simulink model "Sodel_my_6dof_euler"  (R2017b)
settings: Solver=VariableStepAuto  StartTime=0.0  StopTime=Tsim  RelTol=0.01
values from neighbouring files (symbols this model uses):
  u1max = 25*pi/180    (= 0.436332312999)    [init.m]
  u1min = -25*pi/180    (= -0.436332312999)    [init.m]
  u2max = 10*pi/180    (= 0.174532925199)    [init.m]
  u2min = -25*pi/180    (= -0.436332312999)    [init.m]
  u3max = 30*pi/180    (= 0.523598775598)    [init.m]
  u3min = -30*pi/180    (= -0.523598775598)    [init.m]
  u4max = 10*pi/180    (= 0.174532925199)    [init.m]
  u4min = -0.5*pi/180    (= -0.00872664625997)    [init.m]
  u5max = 10*pi/180    (= 0.174532925199)    [init.m]
  u5min = -0.5*pi/180    (= -0.00872664625997)    [init.m]
  uu = [0; -0.1; 0; 0.0821; 0.0821]    [init.m]
  x0 = [100;0;0;0;0;0;0;0.1;0]    [init.m]
undefined symbols (not defined in the file or in its folder): Earth, sodel_6dof, WGS84
libraries: aerolibtransform2 x1, aerolibfltsims x1, shared6dof x1, dspnetwork x1
settings Model: Creator=Admin  LastModifiedBy=Admin
settings ConfigComp: CovHTMLOptions=-sRT=1 -sVT=0 -aTS=1 -bRG=1 -bTC=1 -hTR=1 -nFC=0 -nFD=1 -scm=1 -bcm=1 -xEv=0 -xEM=0

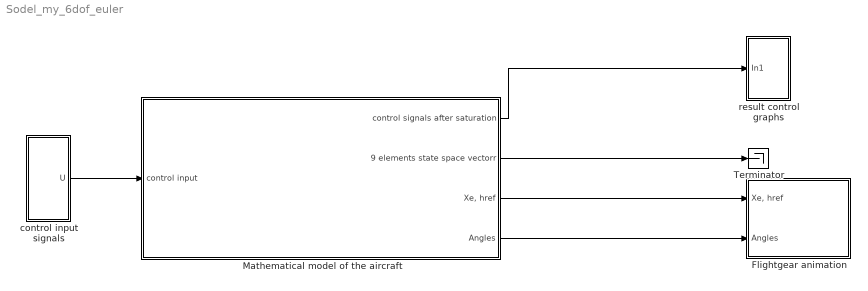
== system Sodel_my_6dof_euler ==
  Flightgear animation : Subsystem
  Mathematical model of the aircraft : Subsystem
  Terminator : Terminator
  control input signals : Subsystem
  result control graphs : Subsystem
  wires:
  control input signals/1(U) -> Mathematical model of the aircraft/1(control input)
  Mathematical model of the aircraft/1(control signals after saturation) -> result control graphs/1(In1)
  Mathematical model of the aircraft/2(9 elements state space vectorr) -> Terminator/1
  Mathematical model of the aircraft/3("Xe, href") -> Flightgear animation/1("Xe, href")
  Mathematical model of the aircraft/4(Angles) -> Flightgear animation/2(Angles)

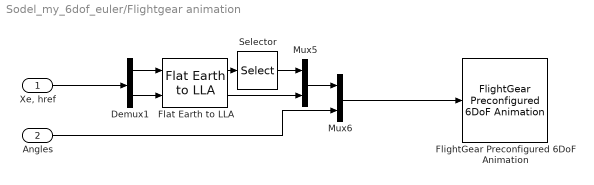
== system Sodel_my_6dof_euler/Flightgear animation ==
  "Xe, href" : Inport
  Angles : Inport  Port=2
  Demux1 : Demux  Outputs=2
  Flat Earth to LLA : aerolibtransform2/Flat Earth to LLA  units=Metric (MKS)  ptype=Earth (WGS84)  F=1/298.257223563  R=6378137  LL0=[37.6272 -122.3896]  psi=0
  FlightGear Preconfigured 6DoF Animation : aerolibfltsims/FlightGear Preconfigured 6DoF Animation  xFlightGearVersion=v2017.1  DestinationIpAddress=127.0.0.1  DestinationPort=5502  SampleTime=1/60
      settings: SourceProductName=Aerospace Blockset
  Mux5 : Mux  Inputs=2
  Mux6 : Mux  Inputs=2
  Selector : Selector  IndexMode=Zero-based  InputPortWidth=2  IndexOptions=Index vector (dialog)  Indices=[1 0]  OutputSizes=1
  wires:
  Mux6/1 -> FlightGear Preconfigured 6DoF Animation/1
  Angles/1 -> Mux6/2
  Demux1/2 -> Flat Earth to LLA/2
  "Xe, href"/1 -> Demux1/1
  Demux1/1 -> Flat Earth to LLA/1
  Flat Earth to LLA/1 -> Selector/1
  Flat Earth to LLA/2 -> Mux5/2
  Selector/1 -> Mux5/1
  Mux5/1 -> Mux6/1

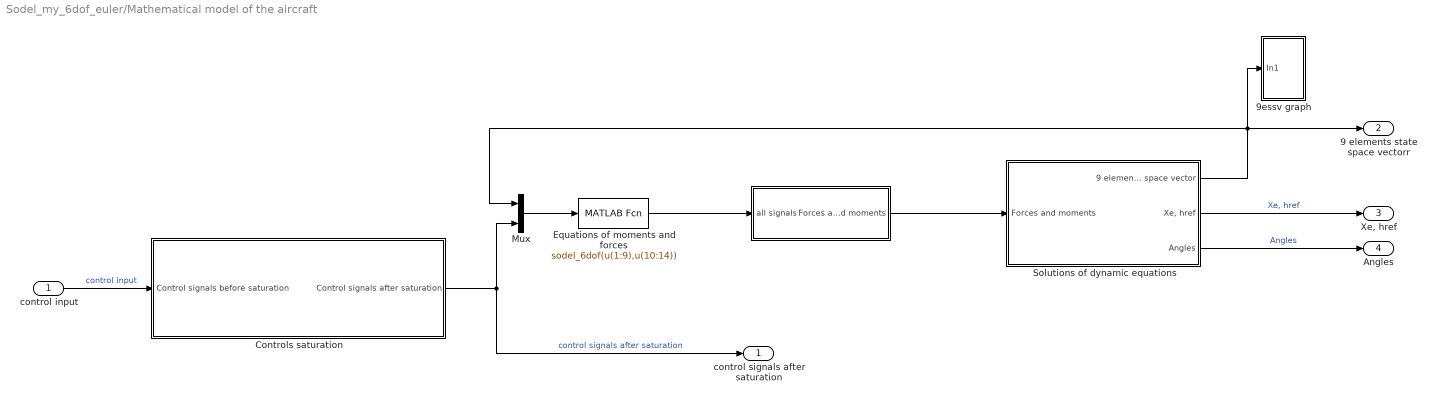
== system Sodel_my_6dof_euler/Mathematical model of the aircraft ==
  control input : Inport
  " " : Subsystem
  9essv graph : Subsystem
  Controls saturation : Subsystem
  Equations of moments and forces : MATLABFcn  MATLABFcn=sodel_6dof(u(1:9),u(10:14))
  Mux : Mux  Inputs=2
  Solutions of dynamic equations : Subsystem
  control signals after saturation : Outport
  9 elements state space vectorr : Outport  Port=2
  "Xe, href" : Outport  Port=3
  Angles : Outport  Port=4
  wires:
  Mux/1 -> Equations of moments and forces/1
  Solutions of dynamic equations/1(9 elements state space vector) -> 9essv graph/1(In1), Mux/1, 9 elements state space vectorr/1
  Solutions of dynamic equations/2("Xe, href") -> "Xe, href"/1  "Xe, href"
  Solutions of dynamic equations/3("Angles ") -> Angles/1  "Angles"
  Controls saturation/1(Control signals after saturation) -> control signals after saturation/1, Mux/2  "control signals after saturation"
  control input/1 -> Controls saturation/1(Control signals before saturation)  "control input"
  Equations of moments and forces/1 -> " "/1("all signals ")
  " "/1(Forces and moments) -> Solutions of dynamic equations/1(Forces and moments)

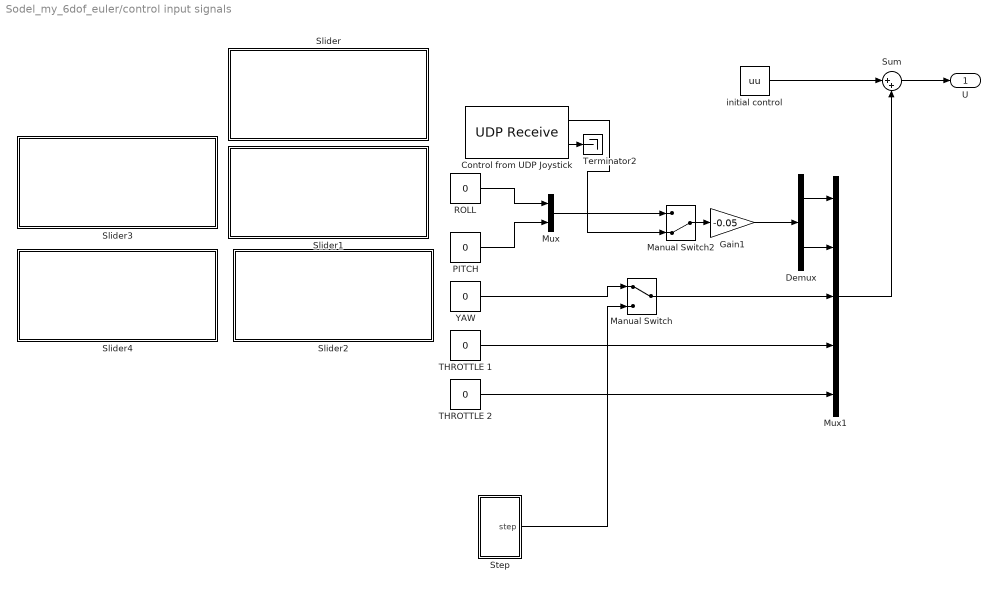
== system Sodel_my_6dof_euler/control input signals ==
  Control from UDP Joystick : dspnetwork/UDP Receive  localURL='0.0.0.0'  localPort=5005  remoteURL='0.0.0.0'  remotePort=-1  recvBufferSize=16  dims=2  signalDatatype=double  isVarSize=off  showBlockingTime=off  blockingTime=0  sampletime=1  blockPlatform=[]
      settings: SourceProductName=DSP System Toolbox  SourceProductBaseCode=DS
  Demux : Demux  Outputs=2
  Gain1 : Gain  Gain=-0.05
  Manual Switch : ManualSwitch
  Manual Switch2 : ManualSwitch  CurrentSetting=0
  Mux : Mux  Inputs=2
  Mux1 : Mux  Inputs=5
  PITCH : Constant  Value=0
  "ROLL " : Constant  Value=0
  Slider : Subsystem  DialogController=hmiCreateDDGDialog  IsWebBlock=on  mask(MWDashboardBlock){webBlockId=4142df3a-b1e0-45a1-953a-8fd48c9debc0, webBlockType=slider, ShowInLibBrowser=on, ShowInitialText=on, HMISrcModelName=Sodel_my_6dof_euler}
      mask prompts: webBlockId "WebBlock Id"; webBlockType "WebBlock Type"; HMISrcModelName "Source Model"
      mask help: SimulinkHMI:dialogs:SliderDialogDesc
      mask Help: helpview([docroot '/mapfiles/simulink.map'], 'hmi_slider')
      mask Display:
      | if strcmp(get_param(bdroot(gcb),'BlockDiagramType'), 'library')
      |     image([(matlabroot) '/toolbox/simulink/hmi/icons/Slider.png']);
      | end
  Slider1 : Subsystem  DialogController=hmiCreateDDGDialog  IsWebBlock=on  mask(MWDashboardBlock){webBlockId=67583dfa-0060-4976-b5ff-87e221de8104, webBlockType=slider, ShowInLibBrowser=on, ShowInitialText=on, HMISrcModelName=Sodel_my_6dof_euler}
      mask prompts: webBlockId "WebBlock Id"; webBlockType "WebBlock Type"; HMISrcModelName "Source Model"
      mask help: SimulinkHMI:dialogs:SliderDialogDesc
      mask Help: helpview([docroot '/mapfiles/simulink.map'], 'hmi_slider')
      mask Display:
      | if strcmp(get_param(bdroot(gcb),'BlockDiagramType'), 'library')
      |     image([(matlabroot) '/toolbox/simulink/hmi/icons/Slider.png']);
      | end
  Slider2 : Subsystem  DialogController=hmiCreateDDGDialog  IsWebBlock=on  mask(MWDashboardBlock){webBlockId=c2c1ebfa-c2dd-4ab2-a502-81d1941be81e, webBlockType=slider, ShowInLibBrowser=on, ShowInitialText=on, HMISrcModelName=Sodel_my_6dof_euler}
      mask prompts: webBlockId "WebBlock Id"; webBlockType "WebBlock Type"; HMISrcModelName "Source Model"
      mask help: SimulinkHMI:dialogs:SliderDialogDesc
      mask Help: helpview([docroot '/mapfiles/simulink.map'], 'hmi_slider')
      mask Display:
      | if strcmp(get_param(bdroot(gcb),'BlockDiagramType'), 'library')
      |     image([(matlabroot) '/toolbox/simulink/hmi/icons/Slider.png']);
      | end
  Slider3 : Subsystem  DialogController=hmiCreateDDGDialog  IsWebBlock=on  mask(MWDashboardBlock){webBlockId=440b1d37-215b-4be1-ba7e-1b8ede8ae161, webBlockType=slider, ShowInLibBrowser=on, ShowInitialText=on, HMISrcModelName=Sodel_my_6dof_euler}
      mask prompts: webBlockId "WebBlock Id"; webBlockType "WebBlock Type"; HMISrcModelName "Source Model"
      mask help: SimulinkHMI:dialogs:SliderDialogDesc
      mask Help: helpview([docroot '/mapfiles/simulink.map'], 'hmi_slider')
      mask Display:
      | if strcmp(get_param(bdroot(gcb),'BlockDiagramType'), 'library')
      |     image([(matlabroot) '/toolbox/simulink/hmi/icons/Slider.png']);
      | end
  Slider4 : Subsystem  DialogController=hmiCreateDDGDialog  IsWebBlock=on  mask(MWDashboardBlock){webBlockId=35d14e88-82ea-4b49-8ecc-39665c181e25, webBlockType=slider, ShowInLibBrowser=on, ShowInitialText=on, HMISrcModelName=Sodel_my_6dof_euler}
      mask prompts: webBlockId "WebBlock Id"; webBlockType "WebBlock Type"; HMISrcModelName "Source Model"
      mask help: SimulinkHMI:dialogs:SliderDialogDesc
      mask Help: helpview([docroot '/mapfiles/simulink.map'], 'hmi_slider')
      mask Display:
      | if strcmp(get_param(bdroot(gcb),'BlockDiagramType'), 'library')
      |     image([(matlabroot) '/toolbox/simulink/hmi/icons/Slider.png']);
      | end
  Step : Subsystem
  Sum : Sum  Inputs=|++
  THROTTLE 1 : Constant  Value=0
  THROTTLE 2 : Constant  Value=0
  Terminator2 : Terminator
  YAW : Constant  Value=0
  initial control : Constant  Value=uu
  U : Outport
  wires:
  Mux1/1 -> Sum/2
  initial control/1 -> Sum/1
  THROTTLE 2/1 -> Mux1/5
  Sum/1 -> U/1
  YAW/1 -> Manual Switch/1
  THROTTLE 1/1 -> Mux1/4
  Manual Switch/1 -> Mux1/3
  Control from UDP Joystick/1 -> Manual Switch2/2
  PITCH/1 -> Mux/2
  "ROLL "/1 -> Mux/1
  Control from UDP Joystick/2 -> Terminator2/1
  Manual Switch2/1 -> Gain1/1
  Demux/1 -> Mux1/1
  Gain1/1 -> Demux/1
  Demux/2 -> Mux1/2
  Mux/1 -> Manual Switch2/1
  Step/1("step ") -> Manual Switch/2

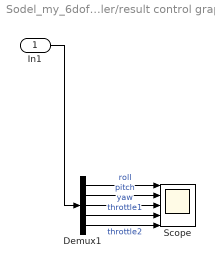
== system Sodel_my_6dof_euler/result control graphs ==
  In1 : Inport
  Demux1 : Demux  Outputs=5
  Scope : Scope  NumInputPorts=5
  wires:
  Demux1/3 -> Scope/3  "yaw"
  Demux1/1 -> Scope/1  "roll"
  Demux1/4 -> Scope/4  "throttle1"
  Demux1/2 -> Scope/2  "pitch"
  Demux1/5 -> Scope/5  "throttle2"
  In1/1 -> Demux1/1

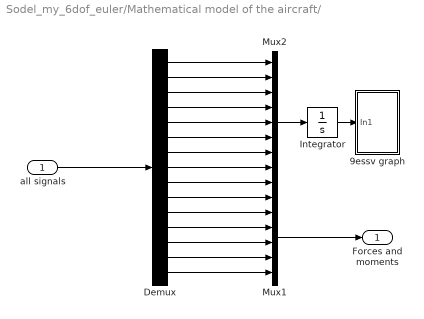
== system Sodel_my_6dof_euler/Mathematical model of the aircraft/  ==
  "all signals " : Inport
  9essv graph : Subsystem
  Demux : Demux  Outputs=15
  Integrator : Integrator  InitialCondition=x0
  Mux1 : Mux  Inputs=6
  Mux2 : Mux  Inputs=9
  Forces and moments : Outport
  wires:
  Mux1/1 -> Forces and moments/1
  Mux2/1 -> Integrator/1
  Demux/8 -> Mux2/8
  Demux/1 -> Mux2/1
  Demux/7 -> Mux2/7
  Demux/13 -> Mux1/4
  Demux/11 -> Mux1/2
  Demux/3 -> Mux2/3
  Demux/4 -> Mux2/4
  Demux/5 -> Mux2/5
  Demux/2 -> Mux2/2
  Demux/10 -> Mux1/1
  Demux/12 -> Mux1/3
  Demux/6 -> Mux2/6
  Demux/15 -> Mux1/6
  Demux/9 -> Mux2/9
  Demux/14 -> Mux1/5
  "all signals "/1 -> Demux/1
  Integrator/1 -> 9essv graph/1(In1)

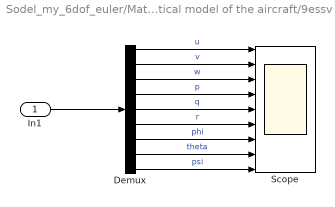
== system Sodel_my_6dof_euler/Mathematical model of the aircraft/9essv graph ==
  In1 : Inport
  Demux : Demux  Outputs=9
  Scope : Scope  NumInputPorts=9
  wires:
  Demux/1 -> Scope/1  "u"
  Demux/2 -> Scope/2  "v"
  Demux/3 -> Scope/3  "w"
  Demux/5 -> Scope/5  "q"
  Demux/4 -> Scope/4  "p"
  Demux/9 -> Scope/9  "psi"
  Demux/8 -> Scope/8  "theta"
  Demux/6 -> Scope/6  "r"
  Demux/7 -> Scope/7  "phi"
  In1/1 -> Demux/1

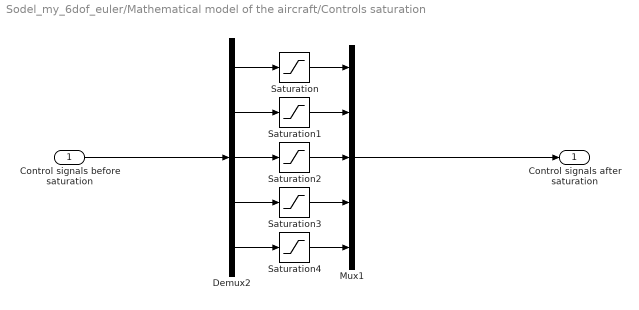
== system Sodel_my_6dof_euler/Mathematical model of the aircraft/Controls saturation ==
  Control signals before saturation : Inport
  Demux2 : Demux  Outputs=5
  Mux1 : Mux  Inputs=5
  Saturation : Saturate  UpperLimit=u1max  LowerLimit=u1min
  Saturation1 : Saturate  UpperLimit=u2max  LowerLimit=u2min
  Saturation2 : Saturate  UpperLimit=u3max  LowerLimit=u3min
  Saturation3 : Saturate  UpperLimit=u4max  LowerLimit=u4min
  Saturation4 : Saturate  UpperLimit=u5max  LowerLimit=u5min
  Control signals after saturation : Outport
  wires:
  Saturation1/1 -> Mux1/2
  Demux2/4 -> Saturation3/1
  Control signals before saturation/1 -> Demux2/1
  Saturation3/1 -> Mux1/4
  Mux1/1 -> Control signals after saturation/1
  Demux2/1 -> Saturation/1
  Demux2/5 -> Saturation4/1
  Saturation2/1 -> Mux1/3
  Saturation/1 -> Mux1/1
  Demux2/3 -> Saturation2/1
  Saturation4/1 -> Mux1/5
  Demux2/2 -> Saturation1/1

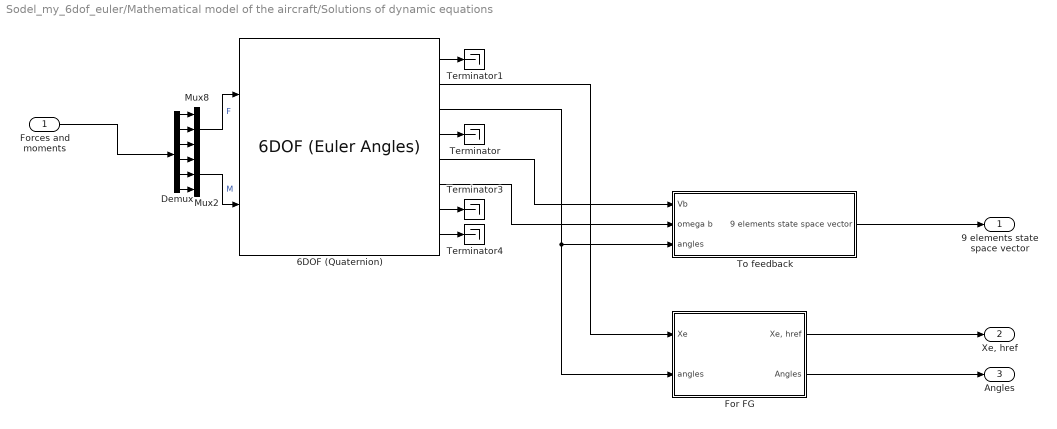
== system Sodel_my_6dof_euler/Mathematical model of the aircraft/Solutions of dynamic equations ==
  Forces and moments : Inport
  6DOF (Quaternion) : shared6dof/6DOF (Euler Angles)  units=Metric (MKS)  mtype=Fixed  rep=Euler Angles  xme_0=[0 0 0]  Vm_0=[100 0 0]  eul_0=[0 0.1 0]  pm_0=[0 0 0]  mass_0=120000  mass_e=0.5  mass_f=2.0  inertia=|  inertia_e=eye(3)  inertia_f=2*eye(3)  k_quat=1.0  vre_flag=on  abi_flag=off
      | 120000*[40.07 0 -2.0923;
      |         0 64 0;
      |         -2.0923 0 99.92]
      settings: SourceProductBaseCode=AE
  Demux : Demux  Outputs=6
  For FG : Subsystem
  Mux2 : Mux  Inputs=3
  Mux8 : Mux  Inputs=3
  Terminator{,1,3..4} (4 alike) : Terminator
  To feedback : Subsystem
  9 elements state space vector : Outport
  "Xe, href" : Outport  Port=2
  "Angles " : Outport  Port=3
  wires:
  6DOF (Quaternion)/2 -> For FG/1(Xe)
  For FG/1("Xe, href") -> "Xe, href"/1
  For FG/2(Angles) -> "Angles "/1
  Demux/6 -> Mux2/3
  Demux/5 -> Mux2/2
  Forces and moments/1 -> Demux/1
  Demux/1 -> Mux8/1
  Demux/2 -> Mux8/2
  Demux/3 -> Mux8/3
  Demux/4 -> Mux2/1
  Mux2/1 -> 6DOF (Quaternion)/2  "M"
  6DOF (Quaternion)/7 -> Terminator3/1
  Mux8/1 -> 6DOF (Quaternion)/1  "F"
  6DOF (Quaternion)/8 -> Terminator4/1
  6DOF (Quaternion)/3 -> To feedback/3(angles), For FG/2(angles)
  6DOF (Quaternion)/4 -> Terminator/1
  6DOF (Quaternion)/1 -> Terminator1/1
  6DOF (Quaternion)/5 -> To feedback/1(Vb)
  6DOF (Quaternion)/6 -> To feedback/2(omega b)
  To feedback/1(9 elements state space vector) -> 9 elements state space vector/1

== system Sodel_my_6dof_euler/control input signals/Slider ==

== system Sodel_my_6dof_euler/control input signals/Slider1 ==

== system Sodel_my_6dof_euler/control input signals/Slider2 ==

== system Sodel_my_6dof_euler/control input signals/Slider3 ==

== system Sodel_my_6dof_euler/control input signals/Slider4 ==

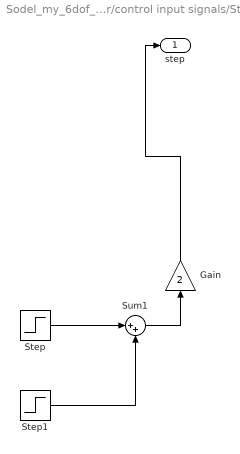
== system Sodel_my_6dof_euler/control input signals/Step ==
  Gain : Gain  Gain=2
  Step : Step  Time=30  After=5*pi/180  SampleTime=0
  Step1 : Step  Time=32  Before=-5*pi/180  After=0  SampleTime=0
  Sum1 : Sum  Inputs=|++
  "step " : Outport
  wires:
  Gain/1 -> "step "/1
  Step1/1 -> Sum1/2
  Step/1 -> Sum1/1
  Sum1/1 -> Gain/1

== system Sodel_my_6dof_euler/Mathematical model of the aircraft/ /9essv graph ==
  In1 : Inport
  Demux : Demux  Outputs=9
  Scope : Scope  NumInputPorts=9
  wires:
  Demux/1 -> Scope/1  "u"
  Demux/2 -> Scope/2  "v"
  Demux/3 -> Scope/3  "w"
  Demux/5 -> Scope/5  "q"
  Demux/4 -> Scope/4  "p"
  Demux/9 -> Scope/9  "psi"
  Demux/8 -> Scope/8  "theta"
  Demux/6 -> Scope/6  "r"
  Demux/7 -> Scope/7  "phi"
  In1/1 -> Demux/1

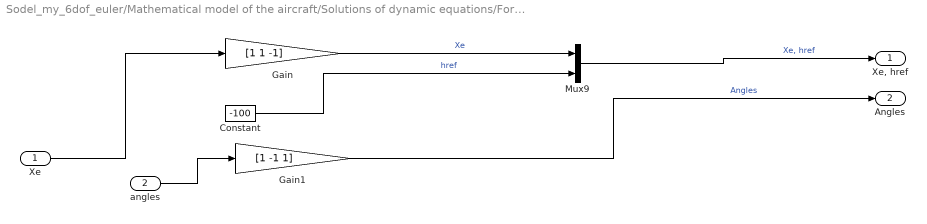
== system Sodel_my_6dof_euler/Mathematical model of the aircraft/Solutions of dynamic equations/For FG ==
  Xe : Inport
  angles : Inport  Port=2
  Constant : Constant  Value=-100
  Gain : Gain  Gain=[1 1 -1]
  Gain1 : Gain  Gain=[1 -1 1]
  Mux9 : Mux  Inputs=2
  "Xe, href" : Outport
  Angles : Outport  Port=2
  wires:
  angles/1 -> Gain1/1
  Mux9/1 -> "Xe, href"/1  "Xe, href"
  Xe/1 -> Gain/1
  Constant/1 -> Mux9/2  "href"
  Gain/1 -> Mux9/1  "Xe"
  Gain1/1 -> Angles/1  "Angles"

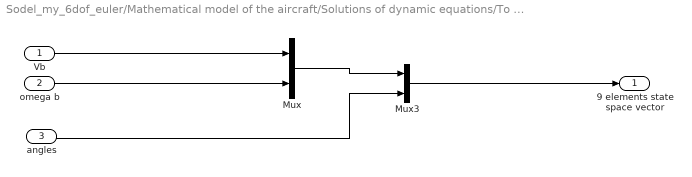
== system Sodel_my_6dof_euler/Mathematical model of the aircraft/Solutions of dynamic equations/To feedback ==
  Vb : Inport
  omega b : Inport  Port=2
  angles : Inport  Port=3
  Mux : Mux  Inputs=2
  Mux3 : Mux  Inputs=2
  9 elements state space vector : Outport
  wires:
  omega b/1 -> Mux/2
  Mux/1 -> Mux3/1
  Vb/1 -> Mux/1
  angles/1 -> Mux3/2
  Mux3/1 -> 9 elements state space vector/1
